simulink model "sim1"  (R2015a)
settings: Solver=ode1  StartTime=0.0  StopTime=15.0  FixedStep=0.1  RelTol=1e-3
settings Model: Creator=Martin  LastModifiedBy=Martin

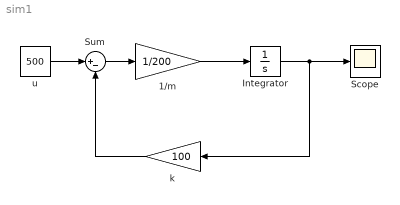
== system sim1 ==
  1/m : Gain  Gain=1/200
  "Integrator " : Integrator
  Scope : Scope
  Sum : Sum  Inputs=|+-
  k : Gain  Gain=100
  u : Constant  Value=500
  wires:
  Sum/1 -> 1/m/1
  1/m/1 -> "Integrator "/1
  "Integrator "/1 -> Scope/1, k/1
  k/1 -> Sum/2
  u/1 -> Sum/1
